simulink model "s16_15"  (R2023b)
settings: Solver=FixedStepDiscrete  StartTime=0.0  StopTime=0  RelTol=1e-3
undefined symbols (not defined in the file or in its folder): strel
libraries: visionmorphops x4, visionsources x3, visiongeotforms x2
settings Model: Creator=lxj  LastModifiedBy=lxj

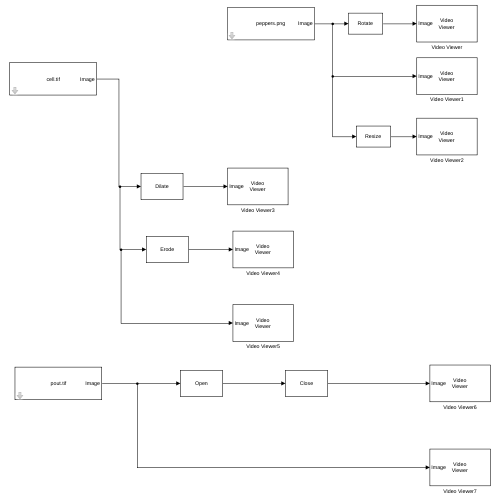
[thumbnail: Simulink's stored preview of the top-level diagram]
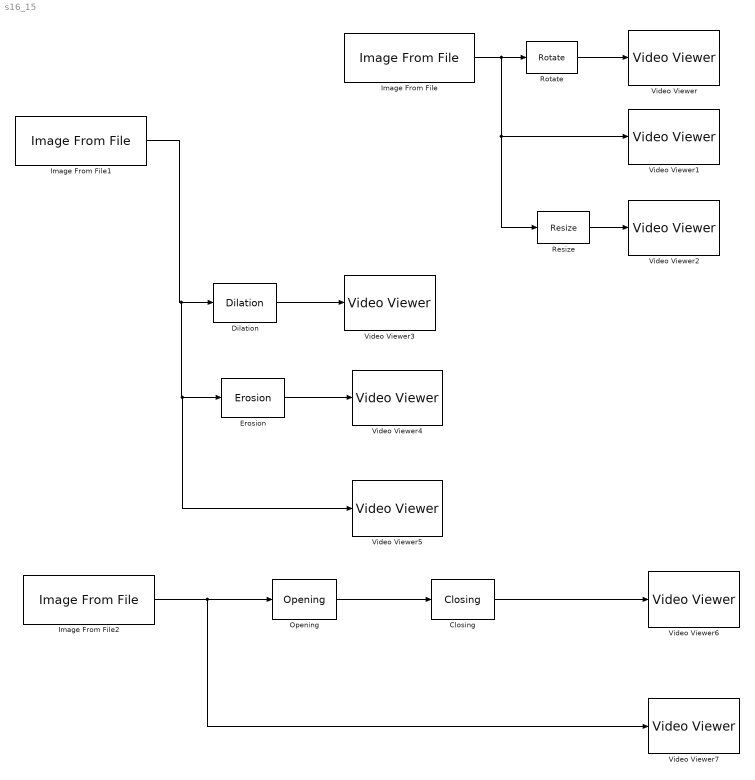
== system s16_15 ==
  Closing : visionmorphops/Closing  nhoodsrc=Specify via dialog  strel=strel('line',5,45)
  Dilation : visionmorphops/Dilation  nhoodsrc=Specify via dialog  strel=[1 1; 1 1]
  Erosion : visionmorphops/Erosion  nhoodsrc=Specify via dialog  strel=strel('square',4)
  Image From File : visionsources/Image From File  Tag=vipblks_nd  FileName=peppers.png  Ts=inf  imagePorts=One multidimensional signal  OutPortLabels=R|G|B  ImageDataType=Inherit from input image  sdImageDataType=uint(8)  Signed=on  WordLength=16  FractionLengthMode=User-defined  FractionLength=15
  Image From File1 : visionsources/Image From File  Tag=vipblks_nd  FileName=cell.tif  Ts=inf  imagePorts=One multidimensional signal  OutPortLabels=R|G|B  ImageDataType=Inherit from input image  sdImageDataType=uint(8)  Signed=on  WordLength=16  FractionLengthMode=User-defined  FractionLength=15
  Image From File2 : visionsources/Image From File  Tag=vipblks_nd  FileName=pout.tif  Ts=inf  imagePorts=One multidimensional signal  OutPortLabels=R|G|B  ImageDataType=Inherit from input image  sdImageDataType=uint(8)  Signed=on  WordLength=16  FractionLengthMode=User-defined  FractionLength=15
  Opening : visionmorphops/Opening  nhoodsrc=Specify via dialog  strel=strel('disk',2)
  Resize : visiongeotforms/Resize  specify=Output size as a percentage of input size  rfactor=[50 50]  outCols=25  outRows=25  outRowsCols=[25 35]  interp_method=Bilinear  antialias=on  useROI=off  roiFlag=off  roundingMode=Nearest  overflowMode=on  prodOutputMode=Binary point scaling  prodOutputWordLength=32  prodOutputFracLength=10
  Rotate : visiongeotforms/Rotate  outSizeR=Expanded to fit rotated input image  src_angle=Specify via dialog  unit_angle=Degrees  angle=pi/4  maxAngle=pi  dispImage=Top-left corner  method=Table lookup  fillVal=0  interpMethod=Bilinear  roundingMode=Nearest  overflowMode=on  prodOutputMode=Binary point scaling  prodOutputWordLength=32  prodOutputFracLength=10
  Video Viewer : VideoViewer  FigPos=[271 695 408 311]
  Video Viewer1 : VideoViewer  FigPos=[605 674 388 325]
  Video Viewer2 : VideoViewer  FigPos=[1113 676 408 311]
  Video Viewer3 : VideoViewer  FigPos=[386 668 408 311]
  Video Viewer4 : VideoViewer  FigPos=[493 662 408 311]
  Video Viewer5 : VideoViewer  FigPos=[1105 665 408 311]
  Video Viewer6 : VideoViewer  FigPos=[332 673 408 311]
  Video Viewer7 : VideoViewer  FigPos=[740 670 408 311]
  wires:
  Rotate/1 -> Video Viewer/1
  Image From File/1 -> Resize/1, Video Viewer1/1, Rotate/1
  Resize/1 -> Video Viewer2/1
  Image From File1/1 -> Video Viewer5/1, Erosion/1, Dilation/1
  Dilation/1 -> Video Viewer3/1
  Erosion/1 -> Video Viewer4/1
  Image From File2/1 -> Video Viewer7/1, Opening/1
  Opening/1 -> Closing/1
  Closing/1 -> Video Viewer6/1
